simulink model "SlidingMode"  (R2025b)
settings: Solver=FixedStepAuto  StartTime=0.0  StopTime=10.0  RelTol=1e-3  EnableMultiTasking=on
undefined symbols (not defined in the file or in its folder): TsControl
libraries: slctrl_smc x1
settings Model: DataDictionary=test.sldd  Creator=rpumpo  LastModifiedBy=rpumpo

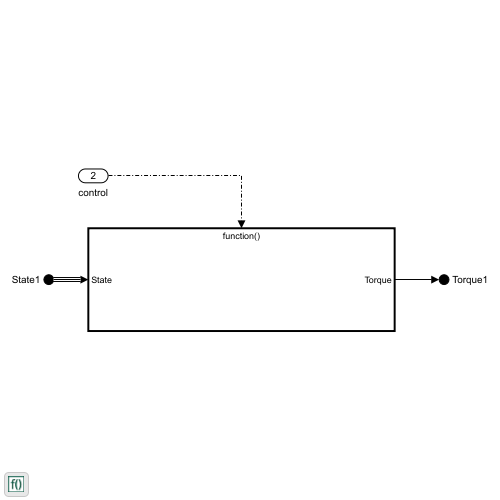
[thumbnail: Simulink's stored preview of the top-level diagram]
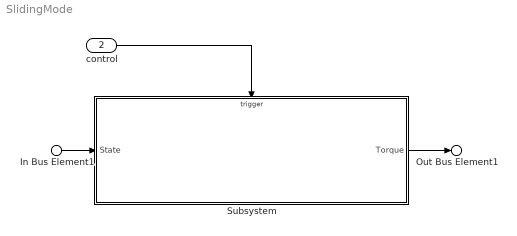
== system SlidingMode ==
  In Bus Element1 : Inport  PortName=State1
  control : Inport  Port=2  SampleTime=TsControl  OutputFunctionCall=on
  Subsystem : Subsystem
  Out Bus Element1 : Outport  PortName=Torque1
  wires:
  control/1 -> Subsystem/Trigger
  Subsystem/1(Torque) -> Out Bus Element1/1
  In Bus Element1/1 -> Subsystem/1(State)

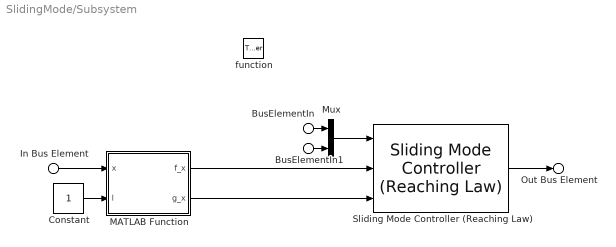
== system SlidingMode/Subsystem ==
  In Bus Element : Inport  PortName=State
  BusElementIn : Inport  PortName=State  Element=position
  BusElementIn1 : Inport  PortName=State  Element=velocity
  function : TriggerPort  TriggerType=function-call  VariantControl=(inherit)
  Constant : Constant
  MATLAB Function : MATLAB Function  TreatAsAtomicUnit=on
  Mux : Mux  Inputs=2
  Sliding Mode Controller (Reaching Law) : slctrl_smc/Sliding Mode Controller (Reaching Law)  TaskMode=Regulation Mode  SlidingMatrix=[0.1 0.1]'  EnableTrackingDerivative=off  EnableSwitchingFunction=off  ReachingLaw=Constant Rate  ReachingRate=0.001  ControlGain=0.01  PowerRate=0.01  BoundaryLayer=Sign  ZeroCross=off  Phi=0.01
  Out Bus Element : Outport  PortName=Torque
  wires:
  BusElementIn/1 -> Mux/1
  Sliding Mode Controller (Reaching Law)/1 -> Out Bus Element/1
  MATLAB Function/2(g_x) -> Sliding Mode Controller (Reaching Law)/3
  BusElementIn1/1 -> Mux/2
  Constant/1 -> MATLAB Function/2(l)
  In Bus Element/1 -> MATLAB Function/1(x)
  MATLAB Function/1(f_x) -> Sliding Mode Controller (Reaching Law)/2
  Mux/1 -> Sliding Mode Controller (Reaching Law)/1

== matlab function SlidingMode/Subsystem/MATLAB Function ==
  data: x input Bus: State; f_x output size=[2 ,1]; l input; g_x output
function [f_x,g_x] = fcn(x,l)
g = 9.81;
f1_x = x.velocity;
f2_x = (g/l)*sin(x.position) ;
f_x = [f1_x, f2_x]';
g_x = [0 , 1]';
